simulink library "NeuroMuscularLibrary"  (R2019b)
settings: Solver=ode45  StartTime=0.0  StopTime=10.0  RelTol=1e-3  EnableMultiTasking=on
values from neighbouring files (symbols this model uses):
  a_18_19 = 116    [Prosthesis3R60Params.m]
  a_18_21 = 34    [Prosthesis3R60Params.m]
  a_2_3 = 18    [Prosthesis3R60Params.m]
  angle_offset = 0    [Prosthesis3R60Params.m]
  ankle_height = 0.08    [BodyMechParams.m]
  c = 0.05    [BodyMechParams.m]
  c_jointstop = 0.3 / (pi/180)    (= 17.1887338539)    [BodyMechParams.m]
  c_stance_comp_a0 = 885.0653    [Prosthesis3R60Params.m]
  c_stance_comp_a1 = 2.1443    [Prosthesis3R60Params.m]
  cg14 = 1/2*L14    (= 0.0475)    [Prosthesis3R60Params.m]
  cg25 = (5.45/11.05)*L25    (= 0.0379527149321)    [Prosthesis3R60Params.m]
  cg3 = (3.6/10.4)*L3    (= 0.0306346153846)    [Prosthesis3R60Params.m]
  d_fBall = 0.1    [BodyMechParams.m]
  d_fHeel = 0.05    [BodyMechParams.m]
  deltaLegAngleThr = 8*pi/180    (= 0.13962634016)    [CMGParams.m]
  DeltaThRef = 2e-3    (= 0.002)    [BodyMechParams.m]
  dt_visual = 0.001    [Prosthesis3R60Params.m]
  eref = 0.04    [BodyMechParams.m]
  Fmax = 4000    [MuscleEnergyTest.m]
  FmaxGLU = 1500    [BodyMechParams.m]
  footBallToAnkleDist = 0.16    [BodyMechParams.m]
  footBallToCenterDist = footLength/2    (= 0.1)    [BodyMechParams.m]
  footBallToHeelDist = footLength    (= 0.2)    [BodyMechParams.m]
  footCenterToCGDist = 0.14 - footBallToCenterDist    (= 0.04)    [BodyMechParams.m]
  footInertia = 0.005    [BodyMechParams.m]
  footLength = 0.2    [BodyMechParams.m]
  footMass = 1.25    [BodyMechParams.m]
  FT = 20    [MuscleEnergyTest.m]
  FT_GLU = 47.6    [BodyMechParams.m]
  g = 9.80665    [BodyMechParams.m]
  groundTheta = [atan(diff(groundZ)./diff(groundX)), 0]    [generateGround.m]
  groundZ = groundZ * stepSize/(largestStep+eps)    [generateGround.m]
  hatCenterToCGDist = 0.35 - hatHipToCenterDistLen    (= -0.05)    [BodyMechParams.m]
  hatHipToCenterDistLen = hatLength/2    (= 0.4)    [BodyMechParams.m]
  hatInertia = 3    [BodyMechParams.m]
  hatLeftHipToCenterDistWidth = .15    (= 0.15)    [BodyMechParams.m]
  hatLength = 0.8    [BodyMechParams.m]
  hatMass = 53.5    [BodyMechParams.m]
  hatThickness = 0.2    [BodyMechParams.m]
  hatWidth = 0.4    [BodyMechParams.m]
  J1011 = (4130)*1e-9    (= 4.13e-06)    [Prosthesis3R60Params.m]
  J1415 = (1.18*1e5)*1e-9    (= 0.000118)    [Prosthesis3R60Params.m]
  J18192021 = (6.86*1e4)*1e-9    (= 6.86e-05)    [Prosthesis3R60Params.m]
  J2526 = (3.59*1e4)*1e-9    (= 3.59e-05)    [Prosthesis3R60Params.m]
  J3467 = (25.96*1e4)*1e-9    (= 0.0002596)    [Prosthesis3R60Params.m]
  K = 5    [BodyMechParams.m]
  k_gn = k_gn/2    (= 39226.6)    [BodyMechParams.m]
  k_gt = k_gt/2    (= 39226.6)    [BodyMechParams.m]
  k_pressure = hatMass * g / DeltaThRef    (= 262327.8875)    [BodyMechParams.m]
  k_stance = 130000    [Prosthesis3R60Params.m]
  k_swing = 18750    [Prosthesis3R60Params.m]
  L0_stance = 0.08925    [Prosthesis3R60Params.m]
  L0_swing = 0.0896    [Prosthesis3R60Params.m]
  L10 = 7.9*1e-3    (= 0.0079)    [Prosthesis3R60Params.m]
  L11 = 3.3*1e-3    (= 0.0033)    [Prosthesis3R60Params.m]
  L14 = 95*1e-3    (= 0.095)    [Prosthesis3R60Params.m]
  L15 = 8.2*1e-3    (= 0.0082)    [Prosthesis3R60Params.m]
  L18 = 25.1*1e-3    (= 0.0251)    [Prosthesis3R60Params.m]
  L19 = 17.7*1e-3    (= 0.0177)    [Prosthesis3R60Params.m]
  L20 = 26*1e-3    (= 0.026)    [Prosthesis3R60Params.m]
  L21 = 1.7*1e-3    (= 0.0017)    [Prosthesis3R60Params.m]
  L25 = 76.95*1e-3    (= 0.07695)    [Prosthesis3R60Params.m]
  L26 = 2.8*1e-3    (= 0.0028)    [Prosthesis3R60Params.m]
  L3 = 88.5*1e-3    (= 0.0885)    [Prosthesis3R60Params.m]
  L4 = 1.7*1e-3    (= 0.0017)    [Prosthesis3R60Params.m]
  L6 = 40.25*1e-3    (= 0.04025)    [Prosthesis3R60Params.m]
  L7 = 14.9*1e-3    (= 0.0149)    [Prosthesis3R60Params.m]
  leg_l = [(thighLength - ankle_height/2) (shankLength - ankle_height/2)]    [BodyMechParams.m]
  legAngleSpeedMax = 10    [CMGParams.m]
  lopt = 0.055    [MuscleEnergyTest.m]
  loptBFSH = 0.12    [BodyMechParams.m]
  loptGAS = 0.05    [BodyMechParams.m]
  loptGLU = 0.11    [BodyMechParams.m]
  loptHAB = 0.09    [BodyMechParams.m]
  loptHAD = 0.10    (= 0.1)    [BodyMechParams.m]
  loptHAM = 0.10    (= 0.1)    [BodyMechParams.m]
  loptHFL = 0.11    [BodyMechParams.m]
  loptRF = 0.08    [BodyMechParams.m]
  loptSOL = 0.04    [BodyMechParams.m]
  loptTA = 0.06    [BodyMechParams.m]
  loptVAS = 0.08    [BodyMechParams.m]
  lslack = 0.245    [MuscleEnergyTest.m]
  lslackBFSH = 0.10    (= 0.1)    [BodyMechParams.m]
  lslackGAS = 0.40    (= 0.4)    [BodyMechParams.m]
  lslackGLU = 0.13    [BodyMechParams.m]
  lslackHAB = 0.07    [BodyMechParams.m]
  lslackHAD = 0.18    [BodyMechParams.m]
  lslackHAM = 0.31    [BodyMechParams.m]
  lslackHFL = 0.10    (= 0.1)    [BodyMechParams.m]
  lslackRF = 0.35    [BodyMechParams.m]
  lslackSOL = 0.26    [BodyMechParams.m]
  lslackTA = 0.24    [BodyMechParams.m]
  lslackVAS = 0.23    [BodyMechParams.m]
  m1011 = 49.5*1e-3    (= 0.0495)    [Prosthesis3R60Params.m]
  m1415 = 123.8*1e-3    (= 0.1238)    [Prosthesis3R60Params.m]
  m18192021 = 196.6*1e-3    (= 0.1966)    [Prosthesis3R60Params.m]
  m2526 = 58.3*1e-3    (= 0.0583)    [Prosthesis3R60Params.m]
  m3467 = 253.3*1e-3    (= 0.2533)    [Prosthesis3R60Params.m]
  mu_slide = 0.8    [BodyMechParams.m]
  mu_stick = 0.9    [BodyMechParams.m]
  N = 1.5    [BodyMechParams.m]    (also in cmaes.m = size(x,1); mergeCompareEnergyCosts.m = {S.name})
  phiKneeUpLimit = 5*pi/180    (= 0.0872664625997)    [BodyMechParams.m]
  phimaxGASa = (100-90)*pi/180    (= 0.174532925199)    [BodyMechParams.m]
  phimaxGASk = (180-140)*pi/180    (= 0.698131700798)    [BodyMechParams.m]
  phimaxRFk = (180-165)*pi/180    (= 0.261799387799)    [BodyMechParams.m]
  phimaxSOL = (100-90)*pi/180    (= 0.174532925199)    [BodyMechParams.m]
  phimaxTA = (80-90)*pi/180    (= -0.174532925199)    [BodyMechParams.m]
  phimaxVAS = (180-165)*pi/180    (= 0.261799387799)    [BodyMechParams.m]
  phirefBFSH = (180-160)*pi/180    (= 0.349065850399)    [BodyMechParams.m]
  phirefGASa = (80-90)*pi/180    (= -0.174532925199)    [BodyMechParams.m]
  phirefGASk = (180-165)*pi/180    (= 0.261799387799)    [BodyMechParams.m]
  phirefGLU = (120-180)*pi/180    (= -1.0471975512)    [BodyMechParams.m]
  phirefHAB = 10*pi/180    (= 0.174532925199)    [BodyMechParams.m]
  phirefHAD = 15*pi/180    (= 0.261799387799)    [BodyMechParams.m]
  phirefHAMh = (150-180)*pi/180    (= -0.523598775598)    [BodyMechParams.m]
  phirefHAMk = (180-180)*pi/180    (= 0)    [BodyMechParams.m]
  phirefHFL = (160-180)*pi/180    (= -0.349065850399)    [BodyMechParams.m]
  phirefRFh = (170-180)*pi/180    (= -0.174532925199)    [BodyMechParams.m]
  phirefRFk = (180-125)*pi/180    (= 0.959931088597)    [BodyMechParams.m]
  phirefSOL = (90-90)*pi/180    (= 0)    [BodyMechParams.m]
  ... (+64 more)
undefined symbols (not defined in the file or in its folder): ankleBackDriveGain, ankleCJointstop, ankleDgain, ankleFilterPID, ankleFilterSEA, ankleGearEff, ankleGearRatio, ankleIgain, ankleInitialAngle, ankleInputMass, ankleIntCoulomb, ankleIntDamping, ankleIntStatic, ankleParallelSpringDamping, ankleParallelSpringOffset, ankleParallelSpringStiffness, anklePgain, anklePlantarLimit, ankleSEADamping, ankleSEAStiffness, ankleTendonMass, ankleWMaxJointstop, D12_F, D12_S, D12_T, D12z_T, D13_F, D1G_F, D1G_HAT, D1G_S, D1G_T, D1Gy_F, DeltaS, DeltaSGLU, DeltaSHFL, dryFrictionDamping, dryFrictionStiffness, dryFrictionVelThresh, footMassp, FourBarL1, FourBarL3, GainDphiHATGLUst, GainDphiHATHABst, GainDphiHATHADst, GainDphiHATHFLst, GainFGASst, GainFGLUst, GainFHABst, GainFHAMst, GainFSOLst, GainFSOLTAst, GainFVASst, GainGAS, GainGLU, GainGLUswing, GainHAM, GainHAMHFL ... (+194)
libraries: sm_lib x332, nesl_utility x156, simulink x33, dspswit3 x30, $bdroot x19, simulink_extras x7
(part 15 of 15)

== system NeuroMuscularLibrary/RMHeel Cnt/3D Contact/Static Friction Model ==
  note: Stiction Limit Detector
  note: Static Friction Model
  note: Zero multiplication prevents
      | horizontal friction model from
      | oscillating between static and kinetic
      | friction when the vertical force is zero but
      | the ground level is not yet reached
      | in the upward motion
  note: (distance to
      | surface)
  note: Tangential Ground Reaction Force
  pos [m] : Inport
  vel [m/s m/s m/s] : Inport  Port=2
  RefPtFP [m m m] : Inport  Port=3
  posFP [m] : Inport  Port=4
  nVecFP [m m m] : Inport  Port=5
  Enable : EnablePort  StatesWhenEnabling=reset  ZeroCross=off
  Abs : Abs
  Check Vertical Friction : Product  RndMeth=Zero
  Constant : Constant
  Dpos_n : DotProduct  InputSameDT=on  OutDataTypeStr=Inherit: Inherit via internal rule
  Dpos_nVec : Product  RndMeth=Zero
  Dpos_tVec : Sum  Inputs=|+-
  FixPt Relational Operator : RelationalOperator  Operator=>  OutDataTypeStr=boolean  ZeroCross=off  RndMeth=Nearest
  Gain : Gain  Gain=-1
  Gain1 : Gain  Gain=k_gn
  Gain2 : Gain  Gain=1/v_gn_max
  Gain3 : Gain  Gain=k_gt
  Gain5 : Gain  Gain=1/v_gt_max
  Memory : Memory
  Mux2 : Mux  Inputs=2
  Normal Ground Reaction Force : Fcn  Expr="u(1)  *  (1-u(2)) * (u(2)<1)"
  Positive : simulink/Logic and Bit Operations/Compare To Zero  relop=>  OutDataTypeStr=boolean
  Positive1 : simulink/Logic and Bit Operations/Compare To Zero  relop=>  OutDataTypeStr=boolean
  Product1 : Product  RndMeth=Zero
  Sign : Signum  ZeroCross=off
  Sum : Sum  Inputs=-+
  Sum1 : Sum  Inputs=|+-
  Sum2 : Sum  Inputs=|+-
  Vector Norm : Subsystem
  d_n : DotProduct  InputSameDT=on  OutDataTypeStr=Inherit: Inherit via internal rule
  stiction limit force : Gain  Gain=mu_stick
  sum : Sum  Inputs=++|
  tVec1 : Product  Inputs=**  RndMeth=Zero
  tVec2 : Product  Inputs=**  RndMeth=Zero
  v_n : DotProduct  InputSameDT=on  OutDataTypeStr=Inherit: Inherit via internal rule
  v_nVec : Product  RndMeth=Zero
  v_tVec : Sum  Inputs=-+|
  F_n Stick [N N N] : Outport  OutputWhenDisabled=reset  InitialOutput=[0 0 0]
      settings: AttributesFormatString=initial = '%<InitialOutput>'\nwhen disabled = '%<OutputWhenDisabled>'
  F_t Stick [N N N] : Outport  Port=2  OutputWhenDisabled=reset  InitialOutput=[0 0 0]
      settings: AttributesFormatString=when disabled: %<OutputWhenDisabled>\ninitial: %<InitialOutput>
  Sliding! : Outport  Port=3  OutputWhenDisabled=reset  InitialOutput=0
      settings: AttributesFormatString=when disabled: %<OutputWhenDisabled>\ninitial: %<InitialOutput>
  wires:
  Sum/1 -> Positive/1
  Memory/1 -> FixPt Relational Operator/2
  Positive/1 -> FixPt Relational Operator/1, Memory/1
  FixPt Relational Operator/1 -> Sliding!/1
  Abs/1 -> Sum/1
  stiction limit force/1 -> Abs/1
  Positive1/1 -> Check Vertical Friction/2
  Check Vertical Friction/1 -> Vector Norm/1(vec), F_t Stick [N N N]/1
  Normal Ground Reaction Force/1 -> Product1/2, stiction limit force/1, Positive1/1
  Mux2/1 -> Normal Ground Reaction Force/1
  Gain1/1 -> Mux2/1
  Gain2/1 -> Mux2/2
  nVecFP [m m m]/1 -> d_n/1, v_n/2, Dpos_n/1, Dpos_nVec/1, v_nVec/2, Product1/1
  d_n/1 -> Gain1/1
  vel [m/s m/s m/s]/1 -> v_tVec/2, v_n/1
  v_n/1 -> v_nVec/1, Gain2/1
  v_nVec/1 -> v_tVec/1
  v_tVec/1 -> Gain5/1
  Product1/1 -> F_n Stick [N N N]/1
  pos [m]/1 -> Sum2/1, Sum1/2
  posFP [m]/1 -> Sum2/2
  Sum2/1 -> Dpos_n/2, Dpos_tVec/1  "Dpos"
  Dpos_n/1 -> Dpos_nVec/2
  Dpos_nVec/1 -> Dpos_tVec/2
  Dpos_tVec/1 -> Gain3/1
  Gain3/1 -> Sign/1, tVec2/2
  Sign/1 -> tVec1/2
  tVec1/1 -> sum/2
  Constant/1 -> sum/1
  sum/1 -> tVec2/1
  tVec2/1 -> Gain/1
  Gain/1 -> Check Vertical Friction/1
  Vector Norm/1(norm) -> Sum/2
  RefPtFP [m m m]/1 -> Sum1/1
  Sum1/1 -> d_n/2
  Gain5/1 -> tVec1/1

== system NeuroMuscularLibrary/Swing Phase (sagittal)/kneeii_damp and hold &kneeiii_leg stop &kneeiv_stance preparation/kneeii_damp and hold ==
  note: Knee Phase ii
  Target Leg Angle : Inport
  VceVAS : Inport  Port=2
  VceBFSH : Inport  Port=3
  VceRF : Inport  Port=4
  LceRF : Inport  Port=5
  Enable : EnablePort  StatesWhenEnabling=reset  ZeroCross=off
  " 1" : Gain  Gain=GainVVASRFsw
  " 2" : Gain  Gain=GainVBFSHsw
  Constant1 : Constant  Value=Sw_a2lopt_RF
  Constant2 : Constant  Value=Sw_aRef_RF
  Constant5 : Constant
  Constant6 : Constant  Value=Sw_phi2lopt_BFSH
  Divide2 : Product  Inputs=3
  Divide3 : Product  Inputs=*/
  Divide4 : Product  Inputs=*/
  Divide6 : Product
  Divide7 : Product  Inputs=*/
  Sum1 : Sum  Inputs=|-+  SaturateOnIntegerOverflow=on  InputSameDT=on  OutDataTypeStr=Inherit: Same as first input
  Sum10 : Sum  Inputs=|++  SaturateOnIntegerOverflow=on  InputSameDT=on  OutDataTypeStr=Inherit: Same as first input
  Sum2 : Sum  Inputs=|-+  SaturateOnIntegerOverflow=on  InputSameDT=on  OutDataTypeStr=Inherit: Same as first input
  Sum7 : Sum  Inputs=|++  SaturateOnIntegerOverflow=on  InputSameDT=on  OutDataTypeStr=Inherit: Same as first input
  positive half{,1..3} (4 alike) : Saturate  UpperLimit=inf  LowerLimit=0  ZeroCross=off
  SRF_Sw_kii : Outport  OutputWhenDisabled=reset  InitialOutput=0
  SBFSH_Sw_kii : Outport  Port=2  OutputWhenDisabled=reset  InitialOutput=0
  wires:
  VceBFSH/1 -> positive half/1, Divide3/1
  " 1"/1 -> SRF_Sw_kii/1
  positive half3/1 -> " 1"/1
  positive half/1 -> " 2"/1
  " 2"/1 -> Divide2/1
  positive half1/1 -> Divide2/2
  VceRF/1 -> Divide4/1
  Constant1/1 -> Divide7/2, Divide6/1, Divide4/2  "a2lopt_RF"
  Sum7/1 -> positive half1/1
  positive half2/1 -> Divide2/3
  Target Leg Angle/1 -> Sum1/2
  Constant2/1 -> Sum1/1  "aRef_RF"
  Sum1/1 -> Divide6/2
  Divide6/1 -> Sum10/1
  Constant5/1 -> Sum10/2
  Sum10/1 -> Sum2/1  "lceOffRF"
  LceRF/1 -> Sum2/2
  Sum2/1 -> Divide7/1
  Divide7/1 -> positive half2/1
  Divide2/1 -> SBFSH_Sw_kii/1
  VceVAS/1 -> positive half3/1
  Divide3/1 -> Sum7/1
  Divide4/1 -> Sum7/2
  Constant6/1 -> Divide3/2

== system NeuroMuscularLibrary/Swing Phase (sagittal)/kneeii_damp and hold &kneeiii_leg stop &kneeiv_stance preparation/kneeiii_leg stop ==
  note: Knee Phase iii
  Target Leg Angle : Inport
  LceHAM : Inport  Port=2
  Enable : EnablePort  StatesWhenEnabling=reset  ZeroCross=off
  " 1" : Gain  Gain=GainSHAMBFSHsw
  " 2" : Gain  Gain=Sw_a2lopt_HAM
  " 3" : Gain  Gain=GainSHAMGASsw
  " 4" : Gain  Gain=GainLHAMsw
  Constant1 : Constant  Value=Sw_aRef_HAM
  Constant2 : Constant  Value=SHAMthresholdsw
  Constant5 : Constant
  Constant6 : Constant  Value=deltaLegAngleThr
  Sum1 : Sum  Inputs=-+|  SaturateOnIntegerOverflow=on  InputSameDT=on  OutDataTypeStr=Inherit: Same as first input
  Sum10 : Sum  Inputs=+-|  SaturateOnIntegerOverflow=on  InputSameDT=on  OutDataTypeStr=Inherit: Same as first input
  Sum2 : Sum  Inputs=|++  SaturateOnIntegerOverflow=on  InputSameDT=on  OutDataTypeStr=Inherit: Same as first input
  Sum3 : Sum  Inputs=-+|  SaturateOnIntegerOverflow=on  InputSameDT=on  OutDataTypeStr=Inherit: Same as first input
  Sum4 : Sum  Inputs=+-|  SaturateOnIntegerOverflow=on  InputSameDT=on  OutDataTypeStr=Inherit: Same as first input
  positive half1 : Saturate  UpperLimit=inf  LowerLimit=0  ZeroCross=off
  positive half2 : Saturate  UpperLimit=inf  LowerLimit=0  ZeroCross=off
  SHAM_Sw_kiii : Outport  OutputWhenDisabled=reset  InitialOutput=0
  SBFSH_Sw_kiii : Outport  Port=2  OutputWhenDisabled=reset  InitialOutput=0
  SGAS_Sw_kiii : Outport  Port=3  OutputWhenDisabled=reset  InitialOutput=0
  wires:
  Sum1/1 -> positive half2/1  "del_LceMAN"
  LceHAM/1 -> Sum1/2  "LceHAM"
  positive half2/1 -> " 4"/1  "del_lce"
  Constant5/1 -> Sum10/1
  " 2"/1 -> Sum10/2
  Target Leg Angle/1 -> Sum2/1
  Sum2/1 -> Sum3/2  "a_thr"
  Sum3/1 -> " 2"/1
  Sum10/1 -> Sum1/1  "lceOffHAM"
  " 4"/1 -> SHAM_Sw_kiii/1, Sum4/1  "S_HAM"
  Sum4/1 -> positive half1/1
  positive half1/1 -> " 1"/1, " 3"/1
  " 1"/1 -> SBFSH_Sw_kiii/1
  " 3"/1 -> SGAS_Sw_kiii/1
  Constant6/1 -> Sum2/2
  Constant1/1 -> Sum3/1
  Constant2/1 -> Sum4/2

== system NeuroMuscularLibrary/Swing Phase (sagittal)/kneeii_damp and hold &kneeiii_leg stop &kneeiv_stance preparation/kneeiv_stance preparation ==
  note: Knee Phase iii
  Target Leg Angle : Inport
  LceHFL : Inport  Port=2
  LceGLU : Inport  Port=3
  LceVAS : Inport  Port=4
  Enable : EnablePort  StatesWhenEnabling=reset  ZeroCross=off
  " 1" : Gain  Gain=GainLGLUsw
  " 2" : Gain  Gain=Sw_phi2lopt_HFL
  " 3" : Gain  Gain=Sw_phi2lopt_GLU
  " 4" : Gain  Gain=GainLHFLsw
  " 5" : Gain  Gain=GainLVASsw
  Constant1 : Constant
  Constant2 : Constant
  Constant4 : Constant  Value=Sw_phiRef_GLU
  Constant5 : Constant  Value=pi/2
  Constant6 : Constant  Value=Sw_phiRef_HFL
  Constant7 : Constant  Value=LceOffsetVASsw
  Sum1 : Sum  Inputs=-+|  SaturateOnIntegerOverflow=on  InputSameDT=on  OutDataTypeStr=Inherit: Same as first input
  Sum2 : Sum  Inputs=++|  SaturateOnIntegerOverflow=on  InputSameDT=on  OutDataTypeStr=Inherit: Same as first input
  Sum3 : Sum  Inputs=|-+  SaturateOnIntegerOverflow=on  InputSameDT=on  OutDataTypeStr=Inherit: Same as first input
  Sum4 : Sum  Inputs=+-|  SaturateOnIntegerOverflow=on  InputSameDT=on  OutDataTypeStr=Inherit: Same as first input
  Sum5 : Sum  Inputs=++|  SaturateOnIntegerOverflow=on  InputSameDT=on  OutDataTypeStr=Inherit: Same as first input
  Sum6 : Sum  Inputs=-+|  SaturateOnIntegerOverflow=on  InputSameDT=on  OutDataTypeStr=Inherit: Same as first input
  Sum7 : Sum  Inputs=+-|  SaturateOnIntegerOverflow=on  InputSameDT=on  OutDataTypeStr=Inherit: Same as first input
  Sum9 : Sum  Inputs=-+|  SaturateOnIntegerOverflow=on  InputSameDT=on  OutDataTypeStr=Inherit: Same as first input
  positive half1 : Saturate  UpperLimit=inf  LowerLimit=0  ZeroCross=off
  positive half2 : Saturate  UpperLimit=inf  LowerLimit=0  ZeroCross=off
  positive half3 : Saturate  UpperLimit=inf  LowerLimit=0  ZeroCross=off
  SHFL_Sw_kiv : Outport  OutputWhenDisabled=reset  InitialOutput=0
  SGLU_Sw_kiv : Outport  Port=2  OutputWhenDisabled=reset  InitialOutput=0
  SVAS_Sw_kiv : Outport  Port=3  OutputWhenDisabled=reset  InitialOutput=0
  wires:
  Sum1/1 -> positive half2/1
  LceHFL/1 -> Sum1/2
  positive half2/1 -> " 4"/1
  Target Leg Angle/1 -> Sum2/2
  Constant5/1 -> Sum2/1
  Sum2/1 -> Sum3/2, Sum4/1
  Sum3/1 -> " 2"/1
  Sum4/1 -> " 3"/1
  " 4"/1 -> SHFL_Sw_kiv/1  "HFL"
  Constant1/1 -> Sum5/1
  " 2"/1 -> Sum5/2
  Sum5/1 -> Sum1/1  "lceOffHFL"
  Sum6/1 -> positive half1/1  "del_lce"
  LceGLU/1 -> Sum6/2  "lceGLU"
  positive half1/1 -> " 1"/1
  " 1"/1 -> SGLU_Sw_kiv/1  "GLU"
  Constant2/1 -> Sum7/1
  " 3"/1 -> Sum7/2
  Sum7/1 -> Sum6/1  "lceOffGLU"
  Sum9/1 -> positive half3/1
  LceVAS/1 -> Sum9/2
  positive half3/1 -> " 5"/1
  " 5"/1 -> SVAS_Sw_kiv/1  "VAS"
  Constant6/1 -> Sum3/1
  Constant4/1 -> Sum4/2
  Constant7/1 -> Sum9/1

== system NeuroMuscularLibrary/Ground Contact Model/2D Contact/Kinetic Friction Model/Vector Norm ==
  vec : Inport
  Constant : Constant  Value=1/2
  Math Function : Math  Operator=pow  SaturateOnIntegerOverflow=on
  Squares : Math  Operator=square  OutputSignalType=real  SaturateOnIntegerOverflow=on
  Sum of Elements : Sum  Inputs=+
  norm : Outport
  wires:
  vec/1 -> Squares/1
  Math Function/1 -> norm/1
  Sum of Elements/1 -> Math Function/1
  Squares/1 -> Sum of Elements/1
  Constant/1 -> Math Function/2

== system NeuroMuscularLibrary/Ground Contact Model/2D Contact/Static Friction Model/Vector Norm ==
  vec : Inport
  Constant : Constant  Value=1/2
  Math Function : Math  Operator=pow  SaturateOnIntegerOverflow=on
  Squares : Math  Operator=square  OutputSignalType=real  SaturateOnIntegerOverflow=on
  Sum of Elements : Sum  Inputs=+
  norm : Outport
  wires:
  vec/1 -> Squares/1
  Math Function/1 -> norm/1
  Sum of Elements/1 -> Math Function/1
  Squares/1 -> Sum of Elements/1
  Constant/1 -> Math Function/2

== system NeuroMuscularLibrary/RMHeel Cnt/3D Contact/Kinetic Friction Model/Vector Norm ==
  vec : Inport
  Constant1 : Constant  Value=.5
  Sqrt : Math  Operator=pow  OutputSignalType=real  SaturateOnIntegerOverflow=on
  Squares : Math  Operator=square  OutputSignalType=real  SaturateOnIntegerOverflow=on
  Sum of Elements : Sum  Inputs=+
  norm : Outport
  wires:
  vec/1 -> Squares/1
  Sqrt/1 -> norm/1
  Sum of Elements/1 -> Sqrt/1
  Squares/1 -> Sum of Elements/1
  Constant1/1 -> Sqrt/2

== system NeuroMuscularLibrary/RMHeel Cnt/3D Contact/Static Friction Model/Vector Norm ==
  vec : Inport
  Constant1 : Constant  Value=.5
  Sqrt : Math  Operator=pow  OutputSignalType=real  SaturateOnIntegerOverflow=on
  Squares : Math  Operator=square  OutputSignalType=real  SaturateOnIntegerOverflow=on
  Sum of Elements : Sum  Inputs=+
  norm : Outport
  wires:
  vec/1 -> Squares/1
  Sqrt/1 -> norm/1
  Sum of Elements/1 -> Sqrt/1
  Squares/1 -> Sum of Elements/1
  Constant1/1 -> Sqrt/2

== stateflow chart NeuroMuscularLibrary/Swing Phase/Chart ==
  settings: updateMethod=CONTINUOUS
  state KneeFlexion
    entry: flex = 1;
    exit: flex = 0;
  state KneeHoldStopAndExtend
    entry: hold = 1;
    exit: hold = 0;
    state KneeStopAndExtend
      entry: stop = 1;
      exit: stop = 0;
      state Extend
        entry: extend = 1;
        exit: extend = 0;
      state KneeStopOnly
      KneeStopOnly -> Extend : [legAngleSpeed >= 0]
      (default) -> KneeStopOnly
    state KneeHoldOnly
    KneeHoldOnly -> KneeStopAndExtend : [(legAngle < (legAngleTgt + ...
        | deltaLegAngleThr)) || Stance]
    (default) -> KneeHoldOnly
  KneeHoldStopAndExtend -> KneeFlexion : [Stance]
  KneeFlexion -> KneeHoldStopAndExtend : [(legLength < legLengthClr) && contraStance && ~Stance]
  (default) -> KneeHoldStopAndExtend
  data: Stance input; contraStance input; deltaLegAngleThr parameter; legAngle input; legAngleSpeed input; legAngleTgt input; legLength input; legLengthClr parameter; flex output double; hold output double; stop output double; extend output double

== stateflow chart NeuroMuscularLibrary/Prosthetic Swing Phase/Chart ==
  settings: updateMethod=CONTINUOUS
  state KneeFlexion
    entry: flex = 1;
    exit: flex = 0;
  state KneeHoldStopAndExtend
    entry: hold = 1;
    exit: hold = 0;
    state KneeStopAndExtend
      entry: stop = 1;
      exit: stop = 0;
      state Extend
        entry: extend = 1;
        exit: extend = 0;
      state KneeStopOnly
      KneeStopOnly -> Extend : [legAngleSpeed >= 0]
      (default) -> KneeStopOnly
    state KneeHoldOnly
    KneeHoldOnly -> KneeStopAndExtend : [(legAngle < (legAngleTgt + ...
        | deltaLegAngleThr)) || Stance]
    (default) -> KneeHoldOnly
  KneeHoldStopAndExtend -> KneeFlexion : [Stance]
  KneeFlexion -> KneeHoldStopAndExtend : [(legLength < legLengthClr) && contraStance && ~Stance]
  (default) -> KneeHoldStopAndExtend
  data: Stance input; contraStance input; deltaLegAngleThr parameter; legAngle input; legAngleSpeed input; legAngleTgt input; legLength input; legLengthClr parameter; flex output double; hold output double; stop output double; extend output double

== matlab function NeuroMuscularLibrary/Otto-bock 3R60/MATLAB Function ==
  data: ICR output; pos14_1 input; pos14_2 input; pos25_1 input; pos25_2 input; alpha output
function [ICR, alpha] = fcn(pos14_1,pos14_2,pos25_1,pos25_2)
ICR = nan(2,1);
alpha = nan(2,1);

y_14_1 = pos14_1(1);
z_14_1 = pos14_1(3);
y_14_2 = pos14_2(1);
z_14_2 = pos14_2(3);
y_25_1 = pos25_1(1);
z_25_1 = pos25_1(3);
y_25_2 = pos25_2(1);
z_25_2 = pos25_2(3);

alpha14 = atan( (z_14_2 - z_14_1)/(y_14_2-y_14_1) );
alpha25 = atan( (z_25_2 - z_25_1)/(y_25_2-y_25_1) );
% origin_swing_y = y_14_2;
% origin_swing_z = z_14_2;
% origin_stance_y = y_14_1;
% origin_stance_z = z_14_1;
% origin_y = origin_stance_y;
% origin_z = origin_stance_z;
%% Swing phase
% line14_z = tand(alpha14)*(y-(y_14_1+origin_swing_y)) + (z_14_1-origin_swing_z);
line14_z = @(y,alpha14)(tan(alpha14)*(y-y_14_1) + z_14_1) ; 
% line14_y = @(z,alpha14)(1/tan(alpha14)*(z-z_14_1) + y_14_1) ; 
% line25_z = @(y,alpha14)(tan(alpha25)*(y-y_25_1) + z_25_1) ; 
% line25_y = @(z,alpha14)(1/tan(alpha25)*(z-z_25_1) + y_25_1) ; 
% line25_z = tand(alpha25-90)*(y-origin_swing_y) + (z_25_1-origin_swing_z);

y = (tan(alpha14)*y_14_1 - z_14_1 - tan(alpha25)*y_25_1 + z_25_1)/(tan(alpha14)-tan(alpha25)); %- origin_swing_y;
% z = (1/tan(alpha14)*z_14_1 -y_14_1 - 1/tan(alpha25)*z_25_1 + y_25_1)/(1/tan(alpha14)-1/tan(alpha25)) - origin_swing_z;
z = line14_z(y,alpha14);
% outy = cos(alpha14)*95*1e-3 + y_14_1;
% 
% outz = sin(alpha14)*95*1e-3 + z_14_1 ;

% outy = line25_y(z_25_2,alpha25) - y_25_2;
% outz = line25_z(y_25_2,alpha25) - z_25_2;

% ICR = [outy; outz];
ICR = [y; z];
alpha = 180/pi.*[alpha14;alpha25];

== matlab function NeuroMuscularLibrary/Detect Gait Phase/MATLAB Function ==
  data: leftLegState_old input; rightLegState_old input; L_GRF input; leftLegState output; rightLegState output; R_GRF input; L_SAGGpos input; R_SAGGpos input; L_norm_foot_shank input; R_norm_foot_shank input
function [leftLegState, rightLegState] = detectGaitPhaseSIM(leftLegState_old, rightLegState_old,L_GRF,R_GRF,L_SAGGpos,R_SAGGpos,L_norm_foot_shank,R_norm_foot_shank)
leftLegState = -9999;
rightLegState = -9999;

[leftLegState, rightLegState] = detectGaitPhase(leftLegState_old, rightLegState_old,L_GRF,R_GRF,L_SAGGpos,R_SAGGpos,L_norm_foot_shank,R_norm_foot_shank);

== stateflow chart NeuroMuscularLibrary/Swing Phase Hip muscle/Chart ==
  settings: updateMethod=CONTINUOUS
  state KneeFlexion
    entry: flex = 1;
    exit: flex = 0;
  state KneeHoldStopAndExtend
    entry: hold = 1;
    exit: hold = 0;
    state KneeStopAndExtend
      entry: stop = 1;
      exit: stop = 0;
      state Extend
        entry: extend = 1;
        exit: extend = 0;
      state KneeStopOnly
      KneeStopOnly -> Extend : [legAngleSpeed >= 0]
      (default) -> KneeStopOnly
    state KneeHoldOnly
    KneeHoldOnly -> KneeStopAndExtend : [(legAngle < (legAngleTgt + ...
        | deltaLegAngleThr)) || Stance]
    (default) -> KneeHoldOnly
  KneeHoldStopAndExtend -> KneeFlexion : [Stance]
  KneeFlexion -> KneeHoldStopAndExtend : [(legLength < legLengthClr) && contraStance && ~Stance]
  (default) -> KneeHoldStopAndExtend
  data: Stance input; contraStance input; deltaLegAngleThr parameter; legAngle input; legAngleSpeed input; legAngleTgt input; legLength input; legLengthClr parameter; flex output double; hold output double; stop output double; extend output double

== matlab function NeuroMuscularLibrary/Otto-Bock Hydraulic Element/MATLAB Function1 ==
  data: x input; F output; dx input
function F = fcn(x,dx)
k = 18750;
x0 = 0.0896;

Fs = -k*(x-x0);
threshold = 0;%1e-5;
if dx < -threshold
    if dx < -20/(60*1000)
        c = (213.5932 * (1/abs(dx)) -4927.5);
    else
        c = 635000/(-20/(60*1000))*dx;
    end
    
%     c = (213.5932 * (1/abs(dx)) -4927.5);
    Fd = -c*dx;
    if Fd < 0
        Fd = 0;
    end
elseif dx > threshold
    if dx > 20/(60*1000)
        c = (146.3288 * (1/abs(dx)) -8808.5);
    else
        c = 429000/(20/(60*1000))*dx;
    end
    
%     c = (146.3288 * (1/abs(dx)) -8808.5);
    Fd = -c*dx;
    if Fd > 0
        Fd = 0;
    end
else
    c = 0;
    Fd = 0;
end

F = Fs + Fd;
